simulink model "Model2_PID"  (R2023b)
settings: Solver=VariableStepAuto  StartTime=0.0  StopTime=6  RelTol=1e-2
values from neighbouring files (symbols this model uses):
  A = pi*((d)^2)/4    (= 0.196349540849)    [Parameters.m]
  a = 2.2*10^-4    (= 0.00022)    [Parameters.m]
  Af = 45    [Parameters.m]
  As = 30    [Parameters.m]
  c = c_*A/L_SMA    (= 0.00981747704247)    [Parameters.m]
  Ca = 10.3    [Parameters.m]
  Cp = 322    [Parameters.m]
  e_l = 0.05    [Parameters.m]
  Ea = 75000    [Parameters.m]
  Em = 28000    [Parameters.m]
  gm = I_max/V_max    (= 0.945945945946)    [Parameters.m]
  h = 36200    [Parameters.m]
  Ip = a*T0/Rp    (= 0.00210434782609)    [Parameters.m]
  k = k_*Ap/t    (= 4.26315789474)    [Parameters.m]
  m = (V*10^-9)/raw    (= 6.08835785579e-12)    [Parameters.m]
  n = 3    [Parameters.m]
  R = 7.8    [Parameters.m]
  R1 = 1000    [Parameters.m]
  R2 = 1000    [Parameters.m]
  R_load = Gv/gm    (= 2.11428571429)    [Parameters.m]
  Rp = 2.3    [Parameters.m]
  T0 = 22    [Parameters.m]
libraries: slpidlib x1
settings Model: Creator=DELL  LastModifiedBy=DELL

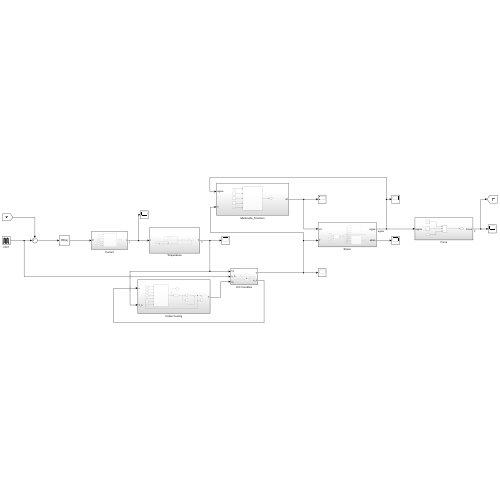
[thumbnail: Simulink's stored preview of the top-level diagram]
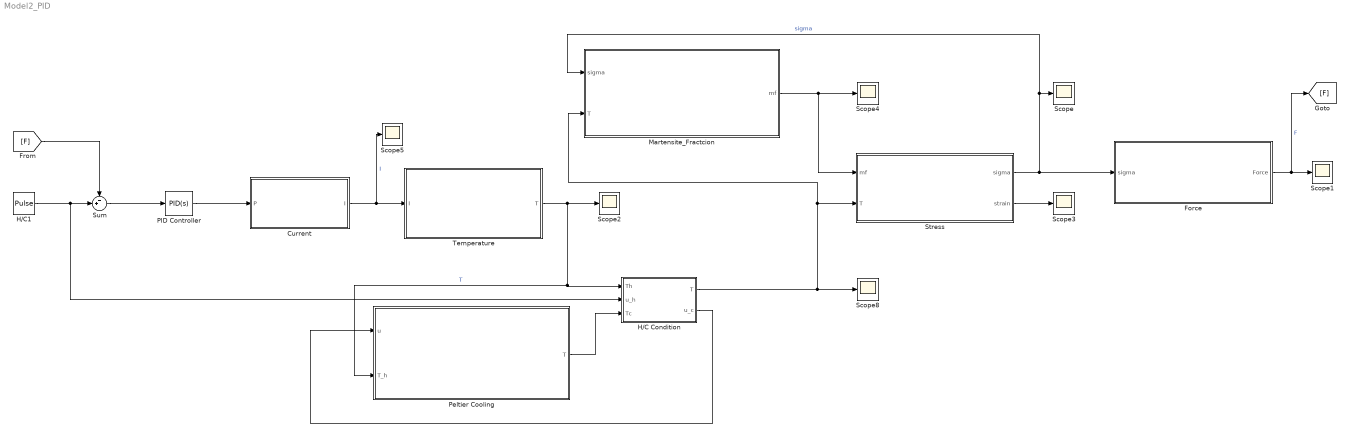
== system Model2_PID ==
  Current : Subsystem
  Force : Subsystem
  H/C Condition : Subsystem
  H/C1 : DiscretePulseGenerator  PulseType=Time based  Amplitude=20  Period=6  PulseWidth=50
  Martensite_Fractcion : Subsystem
  PID Controller : slpidlib/PID Controller  Controller=PID  Form=Parallel  TimeDomain=Continuous-time  UseExternalTs=off  SampleTime=-1  IntegratorMethod=Forward Euler  FilterMethod=Forward Euler  ControllerParametersSource=internal  P=0.00236381141272882  I=7564.45042871426  UseKiTs=off  D=-4.5726759597694e-12  N=516942690.347125  UseFilter=on  TunerSelectOption=Transfer Function Based (PID Tuner App)  InitialConditionSource=internal  InitialConditionForIntegrator=0  InitialConditionForFilter=0  DifferentiatorICPrevScaledInput=0  ExternalReset=none  TrackingMode=off  Kt=1  LimitOutput=off  SatLimitsSource=internal  UpperSaturationLimit=inf  LowerSaturationLimit=-inf  LinearizeAsGain=on  AntiWindupMode=none  Kb=1  LimitIntegrator=off  UpperIntegratorSaturationLimit=inf  LowerIntegratorSaturationLimit=-inf  POutMin=[]  POutMax=[]  IOutMin=[]  IOutMax=[]  DOutMin=[]  DOutMax=[]  NOutMin=[]  NOutMax=[]  SumOutMin=[]  SumOutMax=[]  SaturationOutMin=[]  SaturationOutMax=[]  PParamMin=[]  PParamMax=[]  IParamMin=[]  IParamMax=[]  DParamMin=[]  DParamMax=[]  NParamMin=[]  NParamMax=[]  KbParamMin=[]  KbParamMax=[]  KtParamMin=[]  KtParamMax=[]  KbOutMin=[]  KbOutMax=[]  KtOutMin=[]  KtOutMax=[]  IntegratorOutMin=[]  IntegratorOutMax=[]  FilterOutMin=[]  FilterOutMax=[]  SumI1OutMin=[]  SumI1OutMax=[]  SumI2OutMin=[]  SumI2OutMax=[]  SumI3OutMin=[]  SumI3OutMax=[]  SumI4OutMin=[]  SumI4OutMax=[]  SumDOutMin=[]  SumDOutMax=[]  DifferentiatorOutMin=[]  DifferentiatorOutMax=[]  FilterDiffOutCoefMin=[]  FilterDiffOutCoefMax=[]  ReciprocalOutMin=[]  ReciprocalOutMax=[]  SumDenOutMin=[]  SumDenOutMax=[]  SumNumOutMin=[]  SumNumOutMax=[]  DivideOutMin=[]  DivideOutMax=[]  UdiffTsProdOutMin=[]  UdiffTsProdOutMax=[]  NTsProdOutMin=[]  NTsProdOutMax=[]  UintegralTsProdOutMin=[]  UintegralTsProdOutMax=[]  UngainTsProdOutMin=[]  UngainTsProdOutMax=[]  ClampingZeroOutDataTypeStr=Inherit: Inherit via back propagation  ClampingZeroOutMin=[]  ClampingZeroOutMax=[]  FilterDenConstantOutDataTypeStr=Inherit: Inherit via back propagation  FilterDenConstantOutMin=[]  FilterDenConstantOutMax=[]  PCopyOutDataTypeStr=Inherit: Inherit via back propagation  PCopyOutMin=[]  PCopyOutMax=[]  NCopyOutDataTypeStr=Inherit: Inherit via back propagation  NCopyOutMin=[]  NCopyOutMax=[]  IntegratorContinuousStateAttributes=''  IntegratorStateMustResolveToSignalObject=off  IntegratorRTWStateStorageClass=Auto  FilterContinuousStateAttributes=''  FilterStateMustResolveToSignalObject=off  FilterRTWStateStorageClass=Auto  ParallelPVariant=InternalParameters  IdealPVariant=Disabled  IVariant=InternalParameters  DVariant=InternalParameters  IntegratorVariant=Continuous  SatVariant=Disabled  AWVariant=Passthrough  PCopyVariant=Disabled  TRVariant=Disabled  FdbkBlocksVariant=Forward  IdealPFdbkVariant=Disabled  SatFdbkVariant=Disabled  DerivativeFilterVariant=ContFilter  NVariant=InternalParameters  NCopyVariant=Disabled  FilterICVariant=InternalICsFilter  IntegratorICVariant=InternalICs  ExternalResetVariant=Disabled  TRSumVariant=Passthrough  SumFdbkVariant=Disabled  SumVariant=Sum_PID  TsampFilterVariant=InternalTs  TsampNgainVariant=Passthrough  TsampIntegralVariant=Disabled_SignalSpec  ExternalSaturationOutDataTypeStr=Inherit: Same as second input
  Peltier Cooling : Subsystem
  Scope{,1..5,8} (7 alike) : Scope
  Stress : Subsystem
  Sum : Sum  Inputs=-+|
  Temperature : Subsystem
  wires:
  Martensite_Fractcion/1(mf) -> Scope4/1, Stress/1(mf)
  Stress/1(sigma) -> Martensite_Fractcion/1(sigma), Scope/1, Force/1(sigma)  "sigma"
  Force/1(Force) -> [F], Scope1/1  "F"
  Temperature/1(T) -> Scope2/1, Peltier Cooling/2(T_h), H/C Condition/1(Th)  "T"
  Current/1(I) -> Scope5/1, Temperature/1(I)  "I"
  Stress/2(strain) -> Scope3/1
  H/C Condition/1(T) -> Martensite_Fractcion/2(T), Stress/2(T), Scope8/1
  Peltier Cooling/1(T) -> H/C Condition/3(Tc)
  H/C Condition/2(u_c) -> Peltier Cooling/1(u)
  PID Controller/1 -> Current/1(P)
  Sum/1 -> PID Controller/1
  H/C1/1 -> H/C Condition/2(u_h), Sum/2
  [F] -> Sum/1

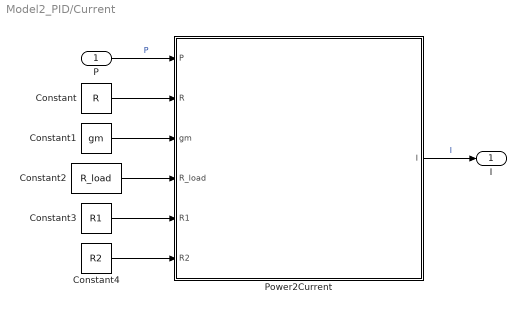
== system Model2_PID/Current ==
  P : Inport
  Constant : Constant  Value=R
  Constant1 : Constant  Value=gm
  Constant2 : Constant  Value=R_load
  Constant3 : Constant  Value=R1
  Constant4 : Constant  Value=R2
  Power2Current : MATLAB Function  TreatAsAtomicUnit=on
  I : Outport
  wires:
  P/1 -> Power2Current/1(P)  "P"
  Power2Current/1(I) -> I/1  "I"
  Constant/1 -> Power2Current/2(R)
  Constant2/1 -> Power2Current/4(R_load)
  Constant3/1 -> Power2Current/5(R1)
  Constant4/1 -> Power2Current/6(R2)
  Constant1/1 -> Power2Current/3(gm)

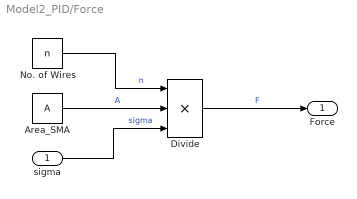
== system Model2_PID/Force ==
  sigma : Inport
  Area_SMA : Constant  Value=A
  Divide : Product  Inputs=***
  No. of Wires : Constant  Value=n
  Force : Outport
  wires:
  Area_SMA/1 -> Divide/2  "A"
  sigma/1 -> Divide/3  "sigma"
  Divide/1 -> Force/1  "F"
  No. of Wires/1 -> Divide/1  "n"

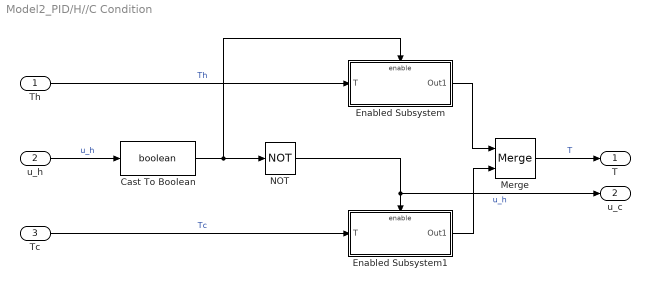
== system Model2_PID/H//C Condition ==
  Th : Inport
  u_h : Inport  Port=2
  Tc : Inport  Port=3
  Cast To Boolean : DataTypeConversion  OutDataTypeStr=boolean  SaturateOnIntegerOverflow=off  RndMeth=Floor
  Enabled Subsystem : Subsystem  TreatAsAtomicUnit=on
  Enabled Subsystem1 : Subsystem  TreatAsAtomicUnit=on
  Merge : Merge
  NOT : Logic  Operator=NOT  IconShape=distinctive  AllPortsSameDT=off  OutDataTypeStr=boolean
  T : Outport
  u_c : Outport  Port=2
  wires:
  Merge/1 -> T/1  "T"
  Enabled Subsystem/1(Out1) -> Merge/1
  Cast To Boolean/1 -> NOT/1, Enabled Subsystem/Enable
  NOT/1 -> u_c/1, Enabled Subsystem1/Enable  "u_h"
  Tc/1 -> Enabled Subsystem1/1(T)  "Tc"
  Th/1 -> Enabled Subsystem/1(T)  "Th"
  Enabled Subsystem1/1(Out1) -> Merge/2
  u_h/1 -> Cast To Boolean/1  "u_h"

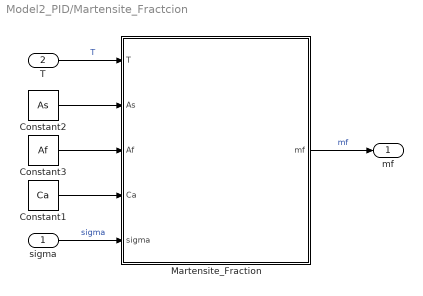
== system Model2_PID/Martensite_Fractcion ==
  sigma : Inport
  T : Inport  Port=2
  Constant1 : Constant  Value=Ca
  Constant2 : Constant  Value=As
  Constant3 : Constant  Value=Af
  Martensite_Fraction : MATLAB Function  TreatAsAtomicUnit=on
  mf : Outport
  wires:
  sigma/1 -> Martensite_Fraction/5(sigma)  "sigma"
  Constant2/1 -> Martensite_Fraction/2(As)
  Martensite_Fraction/1(mf) -> mf/1  "mf"
  T/1 -> Martensite_Fraction/1(T)  "T"
  Constant1/1 -> Martensite_Fraction/4(Ca)
  Constant3/1 -> Martensite_Fraction/3(Af)

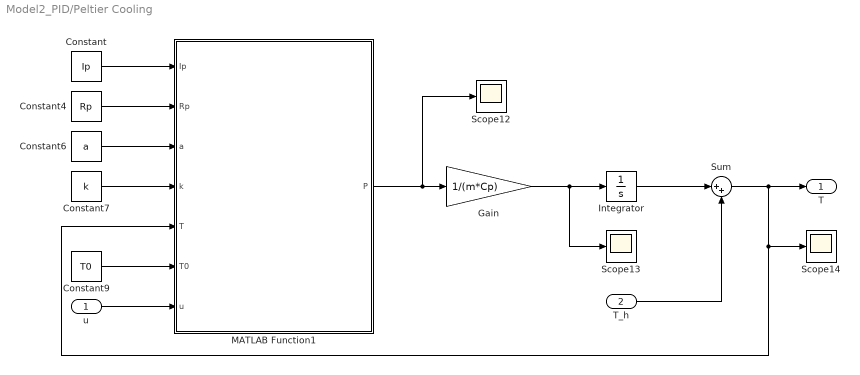
== system Model2_PID/Peltier Cooling ==
  u : Inport
  T_h : Inport  Port=2
  Constant : Constant  Value=Ip
  Constant4 : Constant  Value=Rp
  Constant6 : Constant  Value=a
  Constant7 : Constant  Value=k
  Constant9 : Constant  Value=T0
  Gain : Gain  Gain=1/(m*Cp)
  Integrator : Integrator
  MATLAB Function1 : MATLAB Function  TreatAsAtomicUnit=on
  Scope12 : Scope
  Scope13 : Scope
  Scope14 : Scope
  Sum : Sum  Inputs=|++
  T : Outport
  wires:
  Constant4/1 -> MATLAB Function1/2(Rp)
  MATLAB Function1/1(P) -> Scope12/1, Gain/1
  Constant6/1 -> MATLAB Function1/3(a)
  T_h/1 -> Sum/2
  u/1 -> MATLAB Function1/7(u)
  Constant9/1 -> MATLAB Function1/6(T0)
  Constant/1 -> MATLAB Function1/1(Ip)
  Integrator/1 -> Sum/1
  Sum/1 -> T/1, MATLAB Function1/5(T), Scope14/1
  Gain/1 -> Scope13/1, Integrator/1
  Constant7/1 -> MATLAB Function1/4(k)

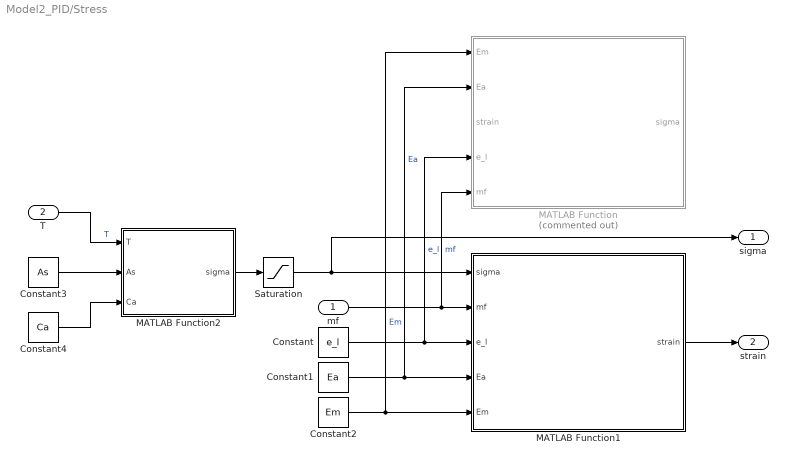
== system Model2_PID/Stress ==
  mf : Inport
  T : Inport  Port=2
  Constant : Constant  Value=e_l
  Constant1 : Constant  Value=Ea
  Constant2 : Constant  Value=Em
  Constant3 : Constant  Value=As
  Constant4 : Constant  Value=Ca
  MATLAB Function : MATLAB Function  Commented=on  TreatAsAtomicUnit=on
  MATLAB Function1 : MATLAB Function  TreatAsAtomicUnit=on
  MATLAB Function2 : MATLAB Function  TreatAsAtomicUnit=on
  Saturation : Saturate  UpperLimit=170  LowerLimit=0
  sigma : Outport
  strain : Outport  Port=2
  wires:
  Constant2/1 -> MATLAB Function/1(Em), MATLAB Function1/5(Em)  "Em"
  Constant1/1 -> MATLAB Function/2(Ea), MATLAB Function1/4(Ea)  "Ea"
  Constant/1 -> MATLAB Function/4(e_l), MATLAB Function1/3(e_l)  "e_l"
  mf/1 -> MATLAB Function/5(mf), MATLAB Function1/2(mf)  "mf"
  MATLAB Function2/1(sigma) -> Saturation/1
  T/1 -> MATLAB Function2/1(T)  "T"
  Constant3/1 -> MATLAB Function2/2(As)
  Constant4/1 -> MATLAB Function2/3(Ca)
  MATLAB Function1/1(strain) -> strain/1
  Saturation/1 -> sigma/1, MATLAB Function1/1(sigma)

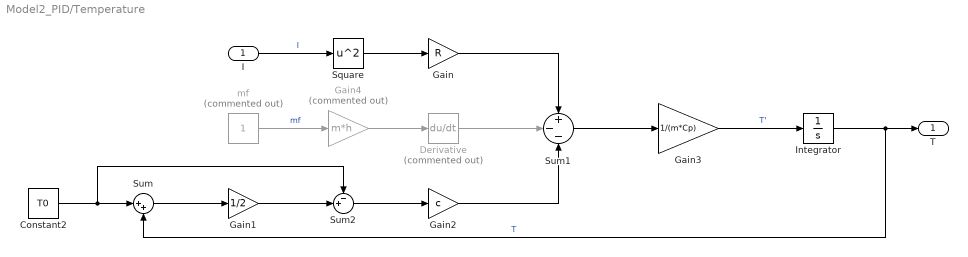
== system Model2_PID/Temperature ==
  I : Inport
  Constant2 : Constant  Value=T0
  Derivative : Derivative  Commented=on
  Gain : Gain  Gain=R
  Gain1 : Gain  Gain=1/2
  Gain2 : Gain  Gain=c
  Gain3 : Gain  Gain=1/(m*Cp)
  Gain4 : Gain  Commented=on  Gain=m*h
  Integrator : Integrator
  Square : Math  Operator=square
  Sum : Sum  Inputs=|++
  Sum1 : Sum  Inputs=+--
  Sum2 : Sum  Inputs=-+|
  mf : Constant  Commented=on
  T : Outport
  wires:
  Gain4/1 -> Derivative/1
  Square/1 -> Gain/1
  Sum1/1 -> Gain3/1
  I/1 -> Square/1  "I"
  Gain/1 -> Sum1/1
  Integrator/1 -> Sum/2, T/1  "T"
  Gain3/1 -> Integrator/1  "T'"
  Derivative/1 -> Sum1/2
  Constant2/1 -> Sum2/1, Sum/1
  Sum/1 -> Gain1/1
  Gain1/1 -> Sum2/2
  Sum2/1 -> Gain2/1
  Gain2/1 -> Sum1/3
  mf/1 -> Gain4/1  "mf"

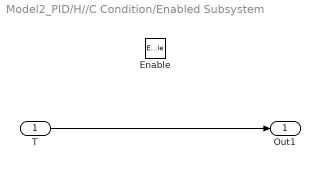
== system Model2_PID/H//C Condition/Enabled Subsystem ==
  T : Inport
  Enable : EnablePort
  Out1 : Outport
  wires:
  T/1 -> Out1/1

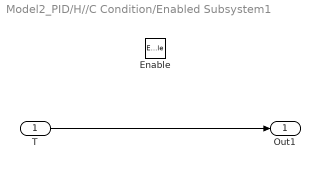
== system Model2_PID/H//C Condition/Enabled Subsystem1 ==
  T : Inport
  Enable : EnablePort
  Out1 : Outport
  wires:
  T/1 -> Out1/1

== matlab function Model2_PID/Martensite_Fractcion/Martensite_Fraction ==
  data: T input; As input; Af input; Ca input; sigma input; mf output
function mf = fcn(T, As, Af, Ca, sigma)

%mf = 1- exp(Ca*(T-As)+Cm*sigma);
%mf = 1- exp(log(0.01)*(As-T)/(As-Af)+sigma*log(0.01)/(Ca*(As-Af)));
if T>As
    mf = 1-(1/2)*(cos(pi*(T-As)/(Af-As)-pi*sigma/(Ca*(Af-As)))+1);
else
    mf = 1;
end

== matlab function Model2_PID/Stress/MATLAB Function ==
  data: Em input; sigma output; Ea input; strain input; e_l input; mf input
function sigma = fcn(Em, Ea, strain, e_l, mf)

E = Em*mf + Ea*(1-mf);

sigma = E*strain - e_l*mf;

== matlab function Model2_PID/Current/Power2Current ==
  data: P input; I output; R input; gm input; R_load input; R1 input; R2 input
function I = fcn(P,R, gm, R_load, R1, R2)

I_req = sqrt(P/R);
V_in = I_req/gm;
Gv = (1+R1/R2);
V_out = V_in*Gv;

I = V_out/R_load;

== matlab function Model2_PID/Stress/MATLAB Function1 ==
  data: sigma input; strain output; mf input; e_l input; Ea input; Em input
function strain = fcn(sigma, mf, e_l, Ea, Em)

E = Em*mf + Ea*(1-mf);

strain = (sigma/E) + e_l*mf;

== matlab function Model2_PID/Stress/MATLAB Function2 ==
  data: T input; sigma output; As input; Ca input
function sigma = fcn(T, As, Ca)

sigma = Ca * (T-As);

== matlab function Model2_PID/Peltier Cooling/MATLAB Function1 ==
  data: Ip input; P output; Rp input; a input; k input; T input; T0 input; u input
function P = fcn(Ip, Rp, a, k, T, T0, u)

Tc = T0;

if (T>T0)&&(u==0)
    I = Ip;
else
    I = 0;
end

P = (1/12)*(I^2)*Rp - a*I*T - k*(T-Tc);
